simulink model "testy"  (R2018a)
settings: Solver=VariableStepAuto  StartTime=0.0  StopTime=10.0  RelTol=1e-3
libraries: sharedTrackingLibrary x1
settings Model: Creator=Zzimon  LastModifiedBy=Zzimon

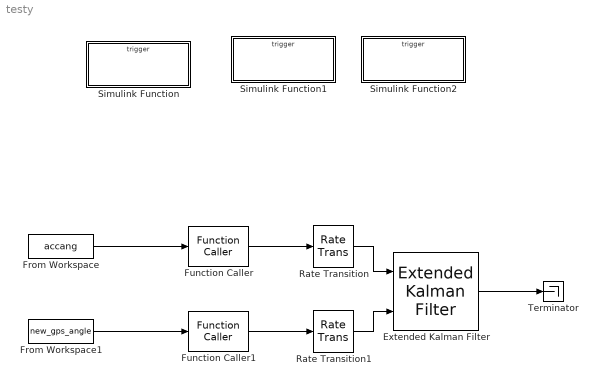
== system testy ==
  Extended Kalman Filter : sharedTrackingLibrary/Extended Kalman Filter  StateTransitionFcn=StateFcn  HasStateTransitionJacobianFcn=off  HasAdditiveProcessNoise=Nonadditive  ProcessNoise=1  HasTimeVaryingProcessNoise=off  HasStateTransitionFcnExtraArgument=0  InitialState=0  InitialStateCovariance=1  MeasurementFcn1=IMU  HasMeasurementJacobianFcn1=off  HasMeasurementEnablePort1=off  HasAdditiveMeasurementNoise1=Additive  MeasurementNoise1=1  HasTimeVaryingMeasurementNoise1=off  HasMeasurementFcnExtraArgument1=0  MeasurementFcn2=GPS  HasMeasurementJacobianFcn2=off  HasMeasurementEnablePort2=off  HasAdditiveMeasurementNoise2=Additive  MeasurementNoise2=1  HasTimeVaryingMeasurementNoise2=off  HasMeasurementFcnExtraArgument2=0  MeasurementFcn3=myMeasurementFcn  HasMeasurementJacobianFcn3=off  HasMeasurementEnablePort3=off  HasAdditiveMeasurementNoise3=Additive  MeasurementNoise3=1  HasTimeVaryingMeasurementNoise3=off  HasMeasurementFcnExtraArgument3=0  MeasurementFcn4=myMeasurementFcn  HasMeasurementJacobianFcn4=off  HasMeasurementEnablePort4=off  HasAdditiveMeasurementNoise4=Additive  MeasurementNoise4=1  HasTimeVaryingMeasurementNoise4=off  HasMeasurementFcnExtraArgument4=0  MeasurementFcn5=myMeasurementFcn  HasMeasurementJacobianFcn5=off  HasMeasurementEnablePort5=off  HasAdditiveMeasurementNoise5=Additive  MeasurementNoise5=1  HasTimeVaryingMeasurementNoise5=off  HasMeasurementFcnExtraArgument5=0  EnableMultirate=off  StateTransitionFcnSampleTime=1  MeasurementFcn1SampleTime=1  MeasurementFcn2SampleTime=1  MeasurementFcn3SampleTime=1  MeasurementFcn4SampleTime=1  MeasurementFcn5SampleTime=1  UseCurrentEstimator=on  OutputStateCovariance=off  DataType=double  SampleTime=1  NumberOfMeasurements=2
      settings: SourceProductName=Control System Toolbox  SourceProductBaseCode=CT
  From Workspace : FromWorkspace  VariableName=accang  SampleTime=0
  From Workspace1 : FromWorkspace  VariableName=new_gps_angle  SampleTime=0
  Function Caller : FunctionCaller  FunctionPrototype=y = IMU(x1)
  Function Caller1 : FunctionCaller  FunctionPrototype=y = GPS(x2)
  Rate Transition : RateTransition
  Rate Transition1 : RateTransition
  Simulink Function : Subsystem  TreatAsAtomicUnit=on
  Simulink Function1 : Subsystem  TreatAsAtomicUnit=on
  Simulink Function2 : Subsystem  TreatAsAtomicUnit=on
  Terminator : Terminator
  wires:
  Rate Transition/1 -> Extended Kalman Filter/1
  Rate Transition1/1 -> Extended Kalman Filter/2
  Extended Kalman Filter/1 -> Terminator/1
  Function Caller/1 -> Rate Transition/1
  Function Caller1/1 -> Rate Transition1/1
  From Workspace/1 -> Function Caller/1
  From Workspace1/1 -> Function Caller1/1

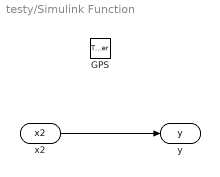
== system testy/Simulink Function ==
  GPS : TriggerPort  TriggerType=function-call  IsSimulinkFunction=on  FunctionName=GPS  FunctionVisibility=scoped  VariantControl=(inherit)
  x2 : ArgIn  DisableCoverage=on  ArgumentName=x2
  y : ArgOut  DisableCoverage=on  ArgumentName=y
  wires:
  x2/1 -> y/1

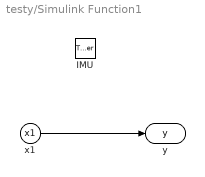
== system testy/Simulink Function1 ==
  IMU : TriggerPort  TriggerType=function-call  IsSimulinkFunction=on  FunctionName=IMU  FunctionVisibility=scoped  VariantControl=(inherit)
  x1 : ArgIn  ArgumentName=x1
  y : ArgOut  DisableCoverage=on  ArgumentName=y
  wires:
  x1/1 -> y/1

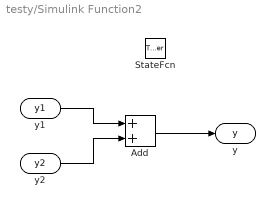
== system testy/Simulink Function2 ==
  StateFcn : TriggerPort  TriggerType=function-call  IsSimulinkFunction=on  FunctionName=StateFcn  FunctionVisibility=scoped  VariantControl=(inherit)
  Add : Sum
  y1 : ArgIn  DisableCoverage=on  ArgumentName=y1
  y2 : ArgIn  Port=2  ArgumentName=y2
  y : ArgOut  DisableCoverage=on  ArgumentName=y
  wires:
  y1/1 -> Add/1
  y2/1 -> Add/2
  Add/1 -> y/1
